simulink model "DealPosLrnd"  (R2018b)
settings: Solver=FixedStepDiscrete  StartTime=0.0  StopTime=10.0  FixedStep=0.01  RelTol=1e-3
undefined symbols (not defined in the file or in its folder): IfKeSMSbSeatMovBkRclnEnable_Val, IfKeSMSbSeatMovBlstOtwdInwdEnable_Val, IfKeSMSbSeatMovCshnFldEnable_Val, IfKeSMSbSeatMovCushnFrtEnable_Val, IfKeSMSbSeatMovFrwdBkwdEnable_Val, IfKeSMSbSeatMovFtrstEnable_Val, IfKeSMSbSeatMovLgrstEnable_Val, IfKeSMSbSeatMovLtwdRtwdEnable_Val, IfVeSMSeStNumConfig, KeSMSbArmscreenMovEnable_Val, KeSMSbIgnorePosLrnd_Val, KeSMSbSeatMovHdFrwdBkwdEnable_Val, KeSMSbSeatMovHdUpwdDnwdEnable_Val, KeSMSbSeatMovLgrstExpdEnable_Val
(part 2 of 2)

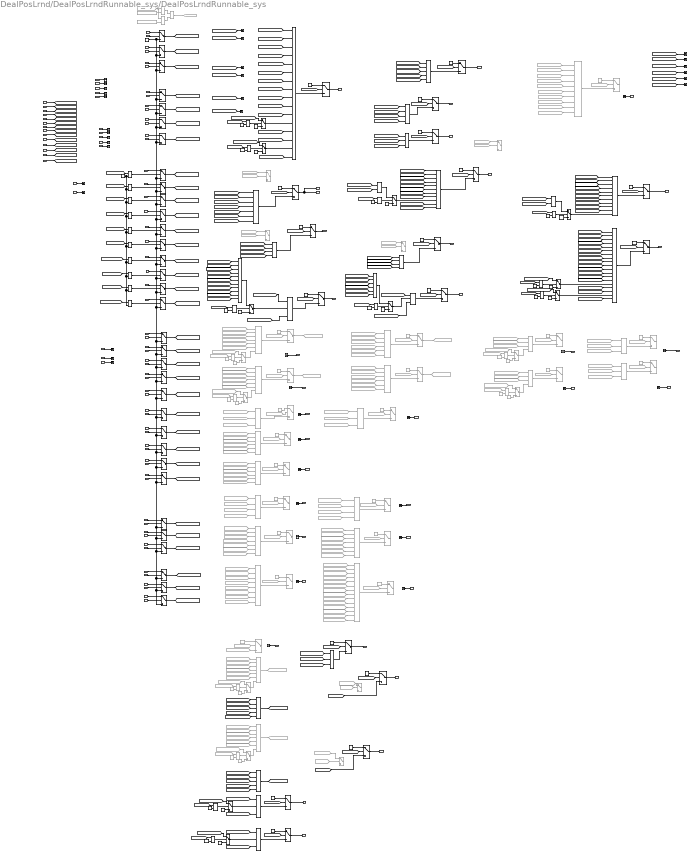
== system DealPosLrnd/DealPosLrndRunnable_sys/DealPosLrndRunnable_sys ==
  note: NOTE:
      | 2023-08-01:新增mode21~26的学习信号，REQ_MSM_607
      | 2023-11-27：四座VIP/全躺/腿托一键打开模式的学习信号，增加前后位置要求。
  note: 四座版本
  note: /* 四座脚踏*/
  note: /*头枕上下*/
  note: /*头枕前后*/
  note: /* 四座腿托伸缩*/
  note: /* 四座脚踏*/
  note: /*头枕前后*/
  note: /* 四座腿托伸缩*/
  note: /*头枕上下*/
  note: 诊断
  note: /*零重力电机*/
  note: /*零重力电机*/
  DrvStBkReclnUpwdDnwdSnsrHmPosLrnd : Inport
  IfVeSMSbDrvStBlstOtwdInwdSnsrHmPosLrnd_Val_read : Inport  Port=2
  IfVeSMSbDrvStCshnFrntUpwdDnwdSnsrHmPosLrnd_Val_read : Inport  Port=3
  IfVeSMSbDrvStCshnRrUpwdDnwdSnsrHmPosLrnd_Val_read : Inport  Port=4
  DrvStFrwdBkwdSnsrHmPosLrnd : Inport  Port=5
  DrvStFtUpwdDnwdSnsrHmPosLrnd : Inport  Port=6
  IfVeSMSbDrvStHdrstUpwdDnwdSnsrHmPosLrnd_Val_read : Inport  Port=7
  IfVeSMSbDrvStLgrstUpwdDnwdSnsrHmPosLrnd_Val_read : Inport  Port=8
  PassStBkReclnUpwdDnwdSnsrHmPosLrnd : Inport  Port=9
  IfVeSMSbPassStBlstOtwdInwdSnsrHmPosLrnd_Val_read : Inport  Port=10
  IfVeSMSbPassStCshnFrntUpwdDnwdSnsrHmPosLrnd_Val_read : Inport  Port=11
  IfVeSMSbPassStCshnRrUpwdDnwdSnsrHmPosLrnd_Val_read : Inport  Port=12
  PassStFrwdBkwdSnsrHmPosLrnd : Inport  Port=13
  PassStFtUpwdDnwdSnsrHmPosLrnd : Inport  Port=14
  IfVeSMSbPassStHdrstUpwdDnwdSnsrHmPosLrnd_Val_read : Inport  Port=15
  IfVeSMSbPassStLgrstUpwdDnwdSnsrHmPosLrnd_Val_read : Inport  Port=16
  SecRwLtStArmScrnSnsrHmPosLrnd : Inport  Port=17
  SecRwLtStBkReclnUpwdDnwdSnsrHmPosLrnd : Inport  Port=18
  SecRwRtStBlstOtwdInwdMovConfig : Inport  Port=19
  IfVeSMSbSecRwLtStBlstOtwdInwdSnsrHmPosLrnd_Val_read : Inport  Port=20
  IfVeSMSbSecRwLtStCshnFrntUpwdDnwdSnsrHmPosLrnd_Val_read : Inport  Port=21
  IfVeSMSbSecRwLtStCshnRrUpwdDnwdSnsrHmPosLrnd_Val_read : Inport  Port=22
  SecRwLtStFrwdBkwdSnsrHmPosLrnd : Inport  Port=23
  SecRwLtStLgrstUpwdDnwdSnsrHmPosLrnd : Inport  Port=24
  SecRwLtStLtwdRtwdSnsrHmPosLrnd : Inport  Port=25
  IfVeSMSbSecRwLtStHdrstUpwdDnwdSnsrHmPosLrnd_Val_read : Inport  Port=26
  IfVeSMSbSecRwRtStArmScrnSnsrHmPosLrnd_Val_read : Inport  Port=27
  SecRwRtStBkReclnUpwdDnwdSnsrHmPosLrnd : Inport  Port=28
  IfVeSMSbSecRwRtStBlstOtwdInwdSnsrHmPosLrnd_Val_read : Inport  Port=29
  IfVeSMSbSecRwRtStCshnFrntUpwdDnwdSnsrHmPosLrnd_Val_read : Inport  Port=30
  IfVeSMSbSecRwRtStCshnRrUpwdDnwdSnsrHmPosLrnd_Val_read : Inport  Port=31
  SecRwRtStFrwdBkwdSnsrHmPosLrnd : Inport  Port=32
  SecRwRtStLgrstUpwdDnwdSnsrHmPosLrnd : Inport  Port=33
  SecRwRtStLtwdRtwdSnsrHmPosLrnd : Inport  Port=34
  IfVeSMSbSecRwRtStHdrstUpwdDnwdSnsrHmPosLrnd_Val_read : Inport  Port=35
  ThdRwLtStBkReclnUpwdDnwdSnsrHmPosLrnd : Inport  Port=36
  ThdRwLtStCshnFldUpwdDnwdSnsrHmPosLrnd : Inport  Port=37
  ThdRwLtStFrwdBkwdSnsrHmPosLrnd : Inport  Port=38
  ThdRwRtStBkReclnUpwdDnwdSnsrHmPosLrnd : Inport  Port=39
  ThdRwRtStCshnFldUpwdDnwdSnsrHmPosLrnd : Inport  Port=40
  ThdRwRtStFrwdBkwdSnsrHmPosLrnd : Inport  Port=41
  KeSMSbSeatMovBkRclnEnable : Inport  Port=42
  KeSMSbSeatMovBlstOtwdInwdEnable : Inport  Port=43
  KeSMSbSeatMovCshnFldEnable : Inport  Port=44
  KeSMSbSeatMovFrwdBkwdEnable : Inport  Port=45
  KeSMSbSeatMovFtrstEnable : Inport  Port=46
  KeSMSbSeatMovLgrstEnable : Inport  Port=47
  KeSMSbSeatMovLtwdRtwdEnable : Inport  Port=48
  KeSMSbIgnorePosLrnd : Inport  Port=49
  KeSMSbArmscreenMovEnable : Inport  Port=50
  DrvStBkReclnUpwdDnwdMovConfig : Inport  Port=51
  DrvStFrwdBkwdMovConfig : Inport  Port=52
  DrvStFtUpwdDnwdMovConfig : Inport  Port=53
  PassStBkReclnUpwdDnwdMovConfig : Inport  Port=54
  PassStFrwdBkwdMovConfig : Inport  Port=55
  PassStFtUpwdDnwdMovConfig : Inport  Port=56
  SecRwRtStBkReclnUpwdDnwdMovConfig : Inport  Port=57
  SecRwRtStFrwdBkwdMovConfig : Inport  Port=58
  SecRwRtStLtwdRtwdMovConfig : Inport  Port=59
  SecRwRtStLgrstUpwdMovConfig : Inport  Port=60
  ThdRwLtStBkReclnUpwdDnwdMovConfig : Inport  Port=61
  ThdRwLtStCshnFldUpwdDnwdMovConfig : Inport  Port=62
  ThdRwLtStFrwdBkwdMovConfig : Inport  Port=63
  ThdRwRtStBkReclnUpwdDnwdMovConfig : Inport  Port=64
  ThdRwRtStCshnFldUpwdDnwdMovConfig : Inport  Port=65
  ThdRwRtStFrwdBkwdMovConfig : Inport  Port=66
  IfVeSMSeStNumConfig : Inport  Port=67
  RrLtStFtUpwdDnwdSnsrHmPosLrnd : Inport  Port=68
  SecRwLtStHdrstFrwdBkwdSnsrHmPosLrnd : Inport  Port=69
  SecRwLtStLgrstOtwdInwdSnsrHmPosLrnd : Inport  Port=70
  RrRtStFtUpwdDnwdSnsrHmPosLrnd : Inport  Port=71
  SecRwRtStHdrstFrwdBkwdSnsrHmPosLrnd : Inport  Port=72
  SecRwRtStLgrstOtwdInwdSnsrHmPosLrnd : Inport  Port=73
  KeSMSbSeatMovHdFrwdBkwdEnable : Inport  Port=74
  KeSMSbSeatMovLgrstExpdEnable : Inport  Port=75
  KeSMSbSeatMovHdUpwdDnwdEnable : Inport  Port=76
  IfVeSMSbRrRtStFtUpwdMovConfig : Inport  Port=77
  IfVeSMSbSecRwRtStHdrstFrwdMovConfig : Inport  Port=78
  IfVeSMSbSecRwRtStLgrstOtwdInwdMovConfig : Inport  Port=79
  IfVeSMSbSecRwRtStHdrstUpwdMovConfig : Inport  Port=80
  IfVeSMSbSecRwRtStArmScrnFrwdBkwdMovConfig : Inport  Port=81
  "IfVeSMSbSecRwRtStCshnFrntUpwdDnwdMovConfig " : Inport  Port=82
  IfKeSMSbSeatMovCushnFrtEnable : Inport  Port=83
  IfVeSMSbPassStFldUpwdDnwdMovConfig : Inport  Port=84
  IfVeSMSbPassStFldUpwdDnwdSnsrHmPosLrnd_Val_read : Inport  Port=85
  AND : Logic  Inputs=16  AllPortsSameDT=off  OutDataTypeStr=boolean
  AND1 : Logic  Commented=on  Inputs=10  AllPortsSameDT=off  OutDataTypeStr=boolean
  AND{6..7,10..11,16,18} (6 alike) : Logic  Inputs=3  AllPortsSameDT=off  OutDataTypeStr=boolean
  AND12 : Logic  AllPortsSameDT=off  OutDataTypeStr=boolean
  AND13 : Logic  Inputs=5  AllPortsSameDT=off  OutDataTypeStr=boolean
  AND14 : Logic  Inputs=11  AllPortsSameDT=off  OutDataTypeStr=boolean
  AND15 : Logic  Inputs=6  AllPortsSameDT=off  OutDataTypeStr=boolean
  AND17 : Logic  Inputs=4  AllPortsSameDT=off  OutDataTypeStr=boolean
  AND19 : Logic  AllPortsSameDT=off  OutDataTypeStr=boolean
  AND2 : Logic  Inputs=7  AllPortsSameDT=off  OutDataTypeStr=boolean
  AND20 : Logic  Inputs=11  AllPortsSameDT=off  OutDataTypeStr=boolean
  AND21 : Logic  Inputs=19  AllPortsSameDT=off  OutDataTypeStr=boolean
  AND3 : Logic  Inputs=11  AllPortsSameDT=off  OutDataTypeStr=boolean
  AND4 : Logic  Inputs=4  AllPortsSameDT=off  OutDataTypeStr=boolean
  AND5 : Logic  Inputs=4  AllPortsSameDT=off  OutDataTypeStr=boolean
  AND8 : Logic  Inputs=5  AllPortsSameDT=off  OutDataTypeStr=boolean
  AND9 : Logic  Inputs=5  AllPortsSameDT=off  OutDataTypeStr=boolean
  Constant{,2..5,13,16,18..19,30,34,37,62..64,67..68} (17 alike) : Constant  Value=true  OutDataTypeStr=boolean
  Constant{1,17,20..24,27..29,40..47,52..53} (20 alike) : Constant  Commented=on  Value=true  OutDataTypeStr=boolean
  Constant{8,10,12,14,26,33,35,66,69,71} (10 alike) : Constant  OutDataTypeStr=uint8
  Constant{7,9,11,25,32,36,65,70,72} (9 alike) : Constant  Value=IfVeSMSeStNumConfig.SeatNum7Config  OutDataTypeStr=Enum: IfVeSMSeStNumConfig
  Constant15 : Constant  Value=IfVeSMSeStNumConfig.SeatNum7Config  OutDataTypeStr=Enum:IfVeSMSeStNumConfig
  Constant31 : Constant  Value=0  OutDataTypeStr=uint8
  Constant38 : Constant  Commented=on  Value=IfVeSMSeStNumConfig.SeatNum4PConfig  OutDataTypeStr=Enum: IfVeSMSeStNumConfig
  Constant39 : Constant  Commented=on  Value=IfVeSMSeStNumConfig.SeatNum4Config  OutDataTypeStr=Enum: IfVeSMSeStNumConfig
  Constant{48,50,54,56,58,60} (6 alike) : Constant  Commented=on  Value=2  OutDataTypeStr=uint8
  Constant{49,51,55,57,59,61} (6 alike) : Constant  Commented=on  OutDataTypeStr=uint8
  Constant6 : Constant  Value=true
  Equal{,1..5,10,25..27} (10 alike) : RelationalOperator  Operator===  OutDataTypeStr=boolean  RndMeth=Simplest
  Equal{6..9,11,13..16,24} (10 alike) : RelationalOperator  Operator=~=  OutDataTypeStr=boolean  RndMeth=Simplest
  Equal{12,17..23} (8 alike) : RelationalOperator  Commented=on  Operator===  OutDataTypeStr=boolean  RndMeth=Simplest
  From{1,11,93,100,109,115,121,164..165,177..178,186,194,202,211,226,234..235,248,252} (20 alike) : From  Commented=on  GotoTag=KeSMSbIgnorePosLrnd
  From{92,101,103,105,131,147} (6 alike) : From  Commented=on  GotoTag=KeSMSeStNum4or4P
  From102 : From  Commented=on  GotoTag=Seat4VIPLtPosLrnd
  From104 : From  Commented=on  GotoTag=Seat4VIPRtPosLrnd
  From106 : From  Commented=on  GotoTag=Seat4RcvyRtPosLrnd
  From{107,112,118,179} (4 alike) : From  Commented=on  GotoTag=SecRwLtStLtwdRtwdSnsrHmPosLrnd
  From{108,114,120,167} (4 alike) : From  Commented=on  GotoTag=SecRwRtStLtwdRtwdSnsrHmPosLrnd
  From110 : From  Commented=on  GotoTag=ThdRwRtStFrwdBkwdSnsrHmPosLrnd
  From{40,111,117,130,166,190,204,213,242,254,258} (11 alike) : From  Commented=on  GotoTag=SecRwLtStFrwdBkwdSnsrHmPosLrnd
  From{45,113,119,168,183,199,208,220,244,256,260} (11 alike) : From  Commented=on  GotoTag=SecRwRtStFrwdBkwdSnsrHmPosLrnd
  From116 : From  Commented=on  GotoTag=ThdRwLtStFrwdBkwdSnsrHmPosLrnd
  From{39,87,124,129,191,203,212,229} (8 alike) : From  Commented=on  GotoTag=SecRwLtStBkReclnUpwdDnwdSnsrHmPosLrnd
  From{41,88,125,174,189,214,230,245} (8 alike) : From  Commented=on  GotoTag=SecRwLtStLgrstUpwdDnwdSnsrHmPosLrnd
  From{89,126,175,188,215,231,246,262} (8 alike) : From  Commented=on  GotoTag=SecRwLtStLgrstOtwdInwdSnsrHmPosLrnd
  From{90,127,176,187,216,232,247} (7 alike) : From  Commented=on  GotoTag=RrLtStFtUpwdDnwdSnsrHmPosLrnd
  From{91,128,139,193,206,218,233} (7 alike) : From  Commented=on  GotoTag=SecRwLtStHdrstUpwdDnwdSnsrHmPosLrnd
  From132 : From  Commented=on  GotoTag=SecRwLtStPosLrnd_Seat4
  From{44,94,134,182,198,207,219,237} (8 alike) : From  Commented=on  GotoTag=SecRwRtStBkReclnUpwdDnwdSnsrHmPosLrnd
  From{46,95,135,171,195,221,238,249} (8 alike) : From  Commented=on  GotoTag=SecRwRtStLgrstUpwdDnwdSnsrHmPosLrnd
  From{96,136,172,197,222,239,250,266} (8 alike) : From  Commented=on  GotoTag=SecRwRtStLgrstOtwdInwdSnsrHmPosLrnd
  From{97,137,173,196,223,240,251} (7 alike) : From  Commented=on  GotoTag=RrRtStFtUpwdDnwdSnsrHmPosLrnd
  From{99,138,185,201,210,225,241} (7 alike) : From  Commented=on  GotoTag=SecRwRtStHdrstUpwdDnwdSnsrHmPosLrnd
  From{140,160,162,192,205,217,228} (7 alike) : From  Commented=on  GotoTag=SecRwLtStHdrstFrwdBkwdSnsrHmPosLrnd
  From148 : From  Commented=on  GotoTag=SecRwRtStPosLrnd_Seat4
  From16 : From  Commented=on  GotoTag=DrvStFtUpwdDnwdSnsrHmPosLrnd
  From{161,163,184,200,209,224,236} (7 alike) : From  Commented=on  GotoTag=SecRwRtStHdrstFrwdBkwdSnsrHmPosLrnd
  From169 : From  Commented=on  GotoTag=ThdRwLtStFrwdBkwdSnsrHmPosLrnd
  From170 : From  Commented=on  GotoTag=ThdRwRtStFrwdBkwdSnsrHmPosLrnd
  From181 : From  Commented=on  GotoTag=IfVeSMSeStNumConfig
  From{227,243,253,255,257,259} (6 alike) : From  Commented=on  GotoTag=KeSMSbSeatMovFrwdBkwdEnable
  From271 : From  Commented=on  GotoTag=SecRwRtStCshnFrntUpwdDnwdSnsrHmPosLrnd
  From49 : From  Commented=on  GotoTag=SecRwLtStCshnFrntUpwdDnwdSnsrHmPosLrnd
  From98 : From  Commented=on  GotoTag=Seat4RcvyLtPosLrnd
  Goto43 : Goto  Commented=on  GotoTag=Seat4VIPLtPosLrnd
  Goto44 : Goto  Commented=on  GotoTag=Seat4VIPRtPosLrnd
  Goto45 : Goto  Commented=on  GotoTag=Seat4RcvyLtPosLrnd
  Goto46 : Goto  Commented=on  GotoTag=Seat4RcvyRtPosLrnd
  Goto47 : Goto  Commented=on  GotoTag=SecRwLtStPosLrnd_Seat4
  Goto49 : Goto  Commented=on  GotoTag=SecRwRtStPosLrnd_Seat4
  Goto51 : Goto  Commented=on  GotoTag=KeSMSeStNum4or4P
  Ground{,5..21} (18 alike) : Ground
  OR{,1,5..6,13..14} (6 alike) : Logic  Commented=on  Inputs=7  AllPortsSameDT=off  OutDataTypeStr=boolean
  OR{2,10,19..20} (4 alike) : Logic  Commented=on  Inputs=3  AllPortsSameDT=off  OutDataTypeStr=boolean
  OR{8..9,11..12} (4 alike) : Logic  Commented=on  Inputs=4  AllPortsSameDT=off  OutDataTypeStr=boolean
  OR15 : Logic  Commented=on  Inputs=8  AllPortsSameDT=off  OutDataTypeStr=boolean
  OR16 : Logic  Commented=on  Inputs=14  AllPortsSameDT=off  OutDataTypeStr=boolean
  OR{3..4,17..18} (4 alike) : Logic  Commented=on  Inputs=6  AllPortsSameDT=off  OutDataTypeStr=boolean
  OR7 : Logic  Commented=on  Operator=OR  AllPortsSameDT=off  OutDataTypeStr=boolean
  Switch{,2..33,35..43,53,55,57..60,64,81..91} (60 alike) : Switch  Criteria=u2 > Threshold
  Switch{1,34,44..52,54,56,61..63,65..80} (32 alike) : Switch  Commented=on  Criteria=u2 > Threshold
  Terminator{,1..26} (27 alike) : Terminator
  IfVeSMSbAcsEntryPosLrnd_Val_write : Outport
  IfVeSMSbAcsExitPosLrnd_Val_write : Outport  Port=2
  IfVeSMSbVIPLtPosLrnd_Val_write : Outport  Port=3
  IfVeSMSbVIPRtPosLrnd_Val_write : Outport  Port=4
  IfVeSMSbRcvyLtPosLrnd_Val_write : Outport  Port=5
  IfVeSMSbRcvyRtPosLrnd_Val_write : Outport  Port=6
  IfVeSMSbLugLtPosLrnd_Val_write : Outport  Port=7
  IfVeSMSbLugRtPosLrnd_Val_write : Outport  Port=8
  IfVeSMSbLyingLtPosLrnd : Outport  Port=9
  IfVeSMSbLyingRtPosLrnd : Outport  Port=10
  IfVeSMSbIntimacyLPosLrnd : Outport  Port=11
  IfVeSMSbFamilyLtPosLrnd : Outport  Port=12
  IfVeSMSbFamilyRtPosLrnd : Outport  Port=13
  IfVeSMSbDrvStPosLrnd_Val_write : Outport  Port=14
  IfVeSMSbPassStPosLrnd_Val_write : Outport  Port=15
  IfVeSMSbSecRwLtStPosLrnd_Val_write : Outport  Port=16
  IfVeSMSbSecRwRtStPosLrnd_Val_write : Outport  Port=17
  IfVeSMSbThdRwLtStPosLrnd_Val_write : Outport  Port=18
  IfVeSMSbThdRwRtStPosLrnd_Val_write : Outport  Port=19
  IfVeSMSbLgrstOpenLtPosLrnd : Outport  Port=20
  IfVeSMSbLgrstCloseLtPosLrnd : Outport  Port=21
  IfVeSMSbLgrstOpenRtPosLrnd : Outport  Port=22
  IfVeSMSbLgrstCloseRtPosLrnd : Outport  Port=23
  IfVeSMSbIntimacyRPosLrnd : Outport  Port=24
  IfVeSMSbAcsEntry4s2LPosLrnd : Outport  Port=25
  IfVeSMSbAcsEntry4s2RPosLrnd : Outport  Port=26
  IfVeSMSbAcsExit4s2LPosLrnd : Outport  Port=27
  IfVeSMSbAcsExit4s2RPosLrnd : Outport  Port=28
  IfVeSMSbAcsEntryAll4sBwdPosLrnd : Outport  Port=29
  IfVeSMSbAcsEntryAll4sFwdPosLrnd : Outport  Port=30
  IfVeSMSbPassReclinerPosLrnd_Val_write : Outport  Port=31
  IfVeSMSbunfold3LPosLrnd_Val_write : Outport  Port=32
  IfVeSMSbunfold3RPosLrnd_Val_write : Outport  Port=33
  IfVeSMSbVIPLtOutPosLrnd_Val_write : Outport  Port=34
  IfVeSMSbVIPRtOutPosLrnd_Val_write : Outport  Port=35
  IfVeSMSbWholeVehMemPosLrnd_Val_write : Outport  Port=36
  wires:
  [KeSMSbIgnorePosLrnd] -> Switch/2
  Switch/1 -> IfVeSMSbAcsEntryPosLrnd_Val_write/1
  Constant/1 -> Switch/1
  From1/1 -> Switch1/2
  Constant1/1 -> Switch1/1
  [KeSMSbIgnorePosLrnd] -> Switch2/2
  Constant2/1 -> Switch2/1
  [KeSMSbIgnorePosLrnd] -> Switch3/2
  Constant3/1 -> Switch3/1
  [KeSMSbIgnorePosLrnd] -> Switch4/2
  Constant4/1 -> Switch4/1
  [KeSMSbIgnorePosLrnd] -> Switch5/2
  Constant5/1 -> Switch5/1
  DrvStBkReclnUpwdDnwdSnsrHmPosLrnd/1 -> Switch6/1
  DrvStFrwdBkwdSnsrHmPosLrnd/1 -> Switch7/1
  DrvStFrwdBkwdMovConfig/1 -> Switch7/2
  DrvStFtUpwdDnwdSnsrHmPosLrnd/1 -> Switch8/1
  PassStBkReclnUpwdDnwdSnsrHmPosLrnd/1 -> Switch9/1
  PassStFrwdBkwdSnsrHmPosLrnd/1 -> Switch10/1
  PassStFtUpwdDnwdSnsrHmPosLrnd/1 -> Switch11/1
  PassStFtUpwdDnwdMovConfig/1 -> Switch11/2
  SecRwLtStBkReclnUpwdDnwdSnsrHmPosLrnd/1 -> Switch12/1
  SecRwLtStFrwdBkwdSnsrHmPosLrnd/1 -> Switch13/1
  SecRwLtStLgrstUpwdDnwdSnsrHmPosLrnd/1 -> Switch14/1
  SecRwLtStLtwdRtwdSnsrHmPosLrnd/1 -> Switch15/1
  SecRwRtStBkReclnUpwdDnwdSnsrHmPosLrnd/1 -> Switch16/1
  SecRwRtStBkReclnUpwdDnwdMovConfig/1 -> Switch16/2
  SecRwRtStFrwdBkwdSnsrHmPosLrnd/1 -> Switch17/1
  SecRwRtStFrwdBkwdMovConfig/1 -> Switch17/2
  SecRwRtStLgrstUpwdMovConfig/1 -> Switch18/2
  SecRwRtStLgrstUpwdDnwdSnsrHmPosLrnd/1 -> Switch18/1
  SecRwRtStLtwdRtwdSnsrHmPosLrnd/1 -> Switch20/1
  SecRwRtStLtwdRtwdMovConfig/1 -> Switch20/2
  ThdRwLtStBkReclnUpwdDnwdSnsrHmPosLrnd/1 -> Switch19/1
  ThdRwLtStBkReclnUpwdDnwdMovConfig/1 -> Switch19/2
  ThdRwLtStCshnFldUpwdDnwdSnsrHmPosLrnd/1 -> Switch21/1
  ThdRwLtStFrwdBkwdSnsrHmPosLrnd/1 -> Switch22/1
  ThdRwRtStBkReclnUpwdDnwdSnsrHmPosLrnd/1 -> Switch23/1
  ThdRwRtStCshnFldUpwdDnwdSnsrHmPosLrnd/1 -> Switch24/1
  ThdRwRtStFrwdBkwdSnsrHmPosLrnd/1 -> Switch25/1
  ThdRwRtStFrwdBkwdMovConfig/1 -> Switch25/2
  KeSMSbSeatMovBkRclnEnable/1 -> [KeSMSbSeatMovBkRclnEnable]
  KeSMSbSeatMovBlstOtwdInwdEnable/1 -> [KeSMSbSeatMovBlstOtwdInwdEnable]
  KeSMSbSeatMovCshnFldEnable/1 -> [KeSMSbSeatMovCshnFldEnable]
  KeSMSbSeatMovFrwdBkwdEnable/1 -> [KeSMSbSeatMovFrwdBkwdEnable]
  KeSMSbSeatMovFtrstEnable/1 -> [KeSMSbSeatMovFtrstEnable]
  KeSMSbSeatMovLgrstEnable/1 -> [KeSMSbSeatMovLgrstEnable]
  KeSMSbSeatMovLtwdRtwdEnable/1 -> [KeSMSbSeatMovLtwdRtwdEnable]
  KeSMSbIgnorePosLrnd/1 -> [KeSMSbIgnorePosLrnd]
  DrvStFtUpwdDnwdMovConfig/1 -> Switch8/2
  PassStBkReclnUpwdDnwdMovConfig/1 -> Switch9/2
  PassStFrwdBkwdMovConfig/1 -> Switch10/2
  ThdRwRtStCshnFldUpwdDnwdMovConfig/1 -> Switch24/2
  IfVeSMSbDrvStLgrstUpwdDnwdSnsrHmPosLrnd_Val_read/1 -> Terminator4/1
  IfVeSMSbDrvStBlstOtwdInwdSnsrHmPosLrnd_Val_read/1 -> Terminator/1
  IfVeSMSbDrvStHdrstUpwdDnwdSnsrHmPosLrnd_Val_read/1 -> Terminator3/1
  IfVeSMSbDrvStCshnFrntUpwdDnwdSnsrHmPosLrnd_Val_read/1 -> Terminator1/1
  IfVeSMSbDrvStCshnRrUpwdDnwdSnsrHmPosLrnd_Val_read/1 -> Terminator2/1
  IfVeSMSbPassStLgrstUpwdDnwdSnsrHmPosLrnd_Val_read/1 -> Terminator9/1
  IfVeSMSbPassStCshnRrUpwdDnwdSnsrHmPosLrnd_Val_read/1 -> Terminator7/1
  IfVeSMSbPassStCshnFrntUpwdDnwdSnsrHmPosLrnd_Val_read/1 -> Terminator6/1
  IfVeSMSbPassStHdrstUpwdDnwdSnsrHmPosLrnd_Val_read/1 -> Terminator8/1
  IfVeSMSbPassStBlstOtwdInwdSnsrHmPosLrnd_Val_read/1 -> Terminator5/1
  IfVeSMSbSecRwLtStBlstOtwdInwdSnsrHmPosLrnd_Val_read/1 -> Terminator11/1
  IfVeSMSbSecRwLtStCshnRrUpwdDnwdSnsrHmPosLrnd_Val_read/1 -> Terminator13/1
  IfVeSMSbSecRwRtStBlstOtwdInwdSnsrHmPosLrnd_Val_read/1 -> Terminator16/1
  IfVeSMSbSecRwRtStCshnRrUpwdDnwdSnsrHmPosLrnd_Val_read/1 -> Terminator18/1
  DrvStBkReclnUpwdDnwdMovConfig/1 -> Switch6/2
  ThdRwLtStCshnFldUpwdDnwdMovConfig/1 -> Switch21/2
  ThdRwLtStFrwdBkwdMovConfig/1 -> Switch22/2
  ThdRwRtStBkReclnUpwdDnwdMovConfig/1 -> Switch23/2
  KeSMSbArmscreenMovEnable/1 -> [KeSMSbArmscreenMovEnable]
  IfVeSMSbSecRwRtStArmScrnSnsrHmPosLrnd_Val_read/1 -> Switch27/1
  SecRwLtStArmScrnSnsrHmPosLrnd/1 -> Switch26/1
  Switch6/1 -> [DrvStBkReclnUpwdDnwdSnsrHmPosLrnd]
  Switch7/1 -> [DrvStFrwdBkwdSnsrHmPosLrnd]
  Switch8/1 -> [DrvStFtUpwdDnwdSnsrHmPosLrnd]
  Switch9/1 -> [PassStBkReclnUpwdDnwdSnsrHmPosLrnd]
  Switch10/1 -> [PassStFrwdBkwdSnsrHmPosLrnd]
  Switch11/1 -> [PassStFtUpwdDnwdSnsrHmPosLrnd]
  Switch12/1 -> [SecRwLtStBkReclnUpwdDnwdSnsrHmPosLrnd]
  Switch13/1 -> [SecRwLtStFrwdBkwdSnsrHmPosLrnd]
  Switch14/1 -> [SecRwLtStLgrstUpwdDnwdSnsrHmPosLrnd]
  Switch15/1 -> [SecRwLtStLtwdRtwdSnsrHmPosLrnd]
  Switch26/1 -> [SecRwLtStArmScrnSnsrHmPosLrnd]
  Switch16/1 -> [SecRwRtStBkReclnUpwdDnwdSnsrHmPosLrnd]
  Switch17/1 -> [SecRwRtStFrwdBkwdSnsrHmPosLrnd]
  Switch18/1 -> [SecRwRtStLgrstUpwdDnwdSnsrHmPosLrnd]
  Switch20/1 -> [SecRwRtStLtwdRtwdSnsrHmPosLrnd]
  Switch27/1 -> [SecRwRtStArmScrnSnsrHmPosLrnd]
  Switch19/1 -> [ThdRwLtStBkReclnUpwdDnwdSnsrHmPosLrnd]
  Switch21/1 -> [ThdRwLtStCshnFldUpwdDnwdSnsrHmPosLrnd]
  Switch22/1 -> [ThdRwLtStFrwdBkwdSnsrHmPosLrnd]
  Switch23/1 -> [ThdRwRtStBkReclnUpwdDnwdSnsrHmPosLrnd]
  Switch24/1 -> [ThdRwRtStCshnFldUpwdDnwdSnsrHmPosLrnd]
  Switch25/1 -> [ThdRwRtStFrwdBkwdSnsrHmPosLrnd]
  IfVeSMSeStNumConfig/1 -> [IfVeSMSeStNumConfig]
  [IfVeSMSeStNumConfig] -> Equal/1
  Constant7/1 -> Equal/2
  Equal/1 -> Switch28/2
  [ThdRwLtStCshnFldUpwdDnwdSnsrHmPosLrnd] -> Switch28/1
  Constant8/1 -> Switch28/3
  Constant10/1 -> Switch29/3
  Equal1/1 -> Switch29/2
  Constant9/1 -> Equal1/2
  [IfVeSMSeStNumConfig] -> Equal1/1
  [ThdRwRtStCshnFldUpwdDnwdSnsrHmPosLrnd] -> Switch29/1
  AND/1 -> Switch/3
  AND1/1 -> Switch1/3
  [SecRwLtStBkReclnUpwdDnwdSnsrHmPosLrnd] -> AND4/1
  [SecRwLtStLgrstUpwdDnwdSnsrHmPosLrnd] -> AND4/2
  [SecRwRtStBkReclnUpwdDnwdSnsrHmPosLrnd] -> AND5/1
  [SecRwRtStLgrstUpwdDnwdSnsrHmPosLrnd] -> AND5/2
  [ThdRwLtStFrwdBkwdSnsrHmPosLrnd] -> AND6/3
  Switch30/1 -> AND6/2
  Constant12/1 -> Switch30/3
  [ThdRwLtStBkReclnUpwdDnwdSnsrHmPosLrnd] -> AND6/1
  Equal2/1 -> Switch30/2
  [IfVeSMSeStNumConfig] -> Equal2/1
  Constant11/1 -> Equal2/2
  Constant13/1 -> Switch31/1
  [KeSMSbIgnorePosLrnd] -> Switch31/2
  AND6/1 -> Switch31/3
  [IfVeSMSeStNumConfig] -> Equal3/1
  Constant15/1 -> Equal3/2
  Equal3/1 -> Switch32/2
  Constant14/1 -> Switch32/3
  Switch32/1 -> AND7/2
  [ThdRwRtStFrwdBkwdSnsrHmPosLrnd] -> AND7/3
  Constant16/1 -> Switch33/1
  [KeSMSbIgnorePosLrnd] -> Switch33/2
  AND7/1 -> Switch33/3
  [ThdRwLtStBkReclnUpwdDnwdSnsrHmPosLrnd] -> AND2/6
  [ThdRwLtStFrwdBkwdSnsrHmPosLrnd] -> AND2/7
  KeSMSbSeatMovHdFrwdBkwdEnable/1 -> [KeSMSbSeatMovHdFrwdBkwdEnable]
  KeSMSbSeatMovLgrstExpdEnable/1 -> [KeSMSbSeatMovLgrstExpdEnable]
  RrLtStFtUpwdDnwdSnsrHmPosLrnd/1 -> Switch36/1
  Switch36/1 -> [RrLtStFtUpwdDnwdSnsrHmPosLrnd]
  IfVeSMSbSecRwLtStHdrstUpwdDnwdSnsrHmPosLrnd_Val_read/1 -> Switch37/1
  Switch37/1 -> [SecRwLtStHdrstUpwdDnwdSnsrHmPosLrnd]
  SecRwLtStHdrstFrwdBkwdSnsrHmPosLrnd/1 -> Switch38/1
  Switch38/1 -> [SecRwLtStHdrstFrwdBkwdSnsrHmPosLrnd]
  SecRwLtStLgrstOtwdInwdSnsrHmPosLrnd/1 -> Switch39/1
  Switch39/1 -> [SecRwLtStLgrstOtwdInwdSnsrHmPosLrnd]
  KeSMSbSeatMovHdUpwdDnwdEnable/1 -> [KeSMSbSeatMovHdUpwdDnwdEnable]
  IfVeSMSbRrRtStFtUpwdMovConfig/1 -> Switch40/2
  RrRtStFtUpwdDnwdSnsrHmPosLrnd/1 -> Switch40/1
  Switch40/1 -> [RrRtStFtUpwdDnwdSnsrHmPosLrnd]
  IfVeSMSbSecRwRtStHdrstFrwdMovConfig/1 -> Switch41/2
  SecRwRtStHdrstFrwdBkwdSnsrHmPosLrnd/1 -> Switch41/1
  Switch41/1 -> [SecRwRtStHdrstFrwdBkwdSnsrHmPosLrnd]
  IfVeSMSbSecRwRtStLgrstOtwdInwdMovConfig/1 -> Switch42/2
  SecRwRtStLgrstOtwdInwdSnsrHmPosLrnd/1 -> Switch42/1
  Switch42/1 -> [SecRwRtStLgrstOtwdInwdSnsrHmPosLrnd]
  IfVeSMSbSecRwRtStHdrstUpwdDnwdSnsrHmPosLrnd_Val_read/1 -> Switch43/1
  Constant6/1 -> Switch7/3, Switch83/3, Switch12/3, Switch13/3, Switch15/3, Switch26/3, Switch36/3, Switch37/3, Switch38/3, Switch39/3, Switch81/3, Switch16/3, Switch17/3, Switch18/3, Switch20/3, Switch27/3, Switch40/3, Switch41/3, Switch42/3, Switch43/3, Switch82/3, Switch23/3, Switch24/3, Switch25/3, Switch22/3, Switch21/3, Switch19/3, Switch14/3, Switch11/3, Switch10/3, Switch9/3, Switch8/3, Switch6/3
  IfVeSMSbSecRwRtStHdrstUpwdMovConfig/1 -> Switch43/2
  Switch43/1 -> [SecRwRtStHdrstUpwdDnwdSnsrHmPosLrnd]
  From87/1 -> OR/1
  From88/1 -> OR/2
  From89/1 -> OR/3
  From90/1 -> OR/4
  From91/1 -> OR/5
  From93/1 -> Switch44/2
  Constant21/1 -> Switch44/1
  OR/1 -> Switch44/3
  Switch44/1 -> Goto43/1
  From94/1 -> OR1/1
  From95/1 -> OR1/2
  From96/1 -> OR1/3
  From97/1 -> OR1/4
  Constant22/1 -> Switch45/1
  From100/1 -> Switch45/2
  OR1/1 -> Switch45/3
  Switch45/1 -> Goto44/1
  From102/1 -> Switch46/1
  From103/1 -> Switch47/2
  From99/1 -> OR1/5
  From104/1 -> Switch47/1
  From98/1 -> Switch48/1
  From105/1 -> Switch49/2
  From106/1 -> Switch49/1
  OR2/1 -> Switch50/3
  From109/1 -> Switch50/2
  Constant27/1 -> Switch50/1
  Constant28/1 -> Switch51/1
  From115/1 -> Switch51/2
  OR3/1 -> Switch51/3
  From121/1 -> Switch52/2
  Constant29/1 -> Switch52/1
  OR4/1 -> Switch52/3
  Switch4/1 -> IfVeSMSbRcvyLtPosLrnd_Val_write/1
  Switch5/1 -> IfVeSMSbRcvyRtPosLrnd_Val_write/1
  From11/1 -> Switch34/2
  Constant17/1 -> Switch34/1
  From16/1 -> Switch34/3
  Constant18/1 -> Switch35/1
  [KeSMSbIgnorePosLrnd] -> Switch35/2
  AND16/1 -> Switch35/3
  [SecRwLtStBkReclnUpwdDnwdSnsrHmPosLrnd] -> AND8/1
  [SecRwLtStFrwdBkwdSnsrHmPosLrnd] -> AND8/2
  [SecRwLtStLgrstUpwdDnwdSnsrHmPosLrnd] -> AND8/3
  [SecRwLtStLgrstOtwdInwdSnsrHmPosLrnd] -> AND8/4
  Constant19/1 -> Switch53/1
  [KeSMSbIgnorePosLrnd] -> Switch53/2
  From125/1 -> OR5/2
  From126/1 -> OR5/3
  From128/1 -> OR5/5
  From124/1 -> OR5/1
  From127/1 -> OR5/4
  AND8/1 -> [SecRwLtStPosLrnd_Seat6_7]
  From132/1 -> Switch54/1
  Switch53/1 -> IfVeSMSbSecRwLtStPosLrnd_Val_write/1
  From134/1 -> OR6/1
  From135/1 -> OR6/2
  From136/1 -> OR6/3
  From137/1 -> OR6/4
  From138/1 -> OR6/5
  OR6/1 -> Goto49/1
  [SecRwRtStCshnFrntUpwdDnwdSnsrHmPosLrnd] -> AND9/5
  [SecRwRtStBkReclnUpwdDnwdSnsrHmPosLrnd] -> AND9/1
  [SecRwRtStFrwdBkwdSnsrHmPosLrnd] -> AND9/2
  [SecRwRtStLgrstUpwdDnwdSnsrHmPosLrnd] -> AND9/3
  [SecRwRtStLgrstOtwdInwdSnsrHmPosLrnd] -> AND9/4
  AND9/1 -> [SecRwRtStPosLrnd_Seat6_7]
  [KeSMSbIgnorePosLrnd] -> Switch55/2
  Constant30/1 -> Switch55/1
  From148/1 -> Switch56/1
  From147/1 -> Switch56/2
  Switch55/1 -> IfVeSMSbSecRwRtStPosLrnd_Val_write/1
  Constant33/1 -> Switch57/3
  [ThdRwLtStCshnFldUpwdDnwdSnsrHmPosLrnd] -> Switch57/1
  Equal5/1 -> Switch57/2
  [IfVeSMSeStNumConfig] -> Equal5/1
  Constant32/1 -> Equal5/2
  Constant34/1 -> Switch58/1
  AND10/1 -> Switch58/3
  [KeSMSbIgnorePosLrnd] -> Switch58/2
  [ThdRwLtStBkReclnUpwdDnwdSnsrHmPosLrnd] -> AND10/1
  Switch57/1 -> AND10/2
  [ThdRwLtStFrwdBkwdSnsrHmPosLrnd] -> AND10/3
  Switch58/1 -> IfVeSMSbThdRwLtStPosLrnd_Val_write/1
  Constant36/1 -> Equal10/2
  Equal10/1 -> Switch59/2
  [IfVeSMSeStNumConfig] -> Equal10/1
  [ThdRwRtStCshnFldUpwdDnwdSnsrHmPosLrnd] -> Switch59/1
  Constant35/1 -> Switch59/3
  [ThdRwRtStBkReclnUpwdDnwdSnsrHmPosLrnd] -> AND11/1
  [ThdRwRtStFrwdBkwdSnsrHmPosLrnd] -> AND11/3
  Switch59/1 -> AND11/2
  [KeSMSbIgnorePosLrnd] -> Switch60/2
  Constant37/1 -> Switch60/1
  AND11/1 -> Switch60/3
  Switch60/1 -> IfVeSMSbThdRwRtStPosLrnd_Val_write/1
  OR5/1 -> Goto47/1
  From160/1 -> OR/6
  From161/1 -> OR1/6
  From162/1 -> OR5/6
  From163/1 -> OR6/6
  Constant38/1 -> Equal17/2
  OR7/1 -> Goto51/1
  Equal17/1 -> OR7/2
  Constant39/1 -> Equal12/2
  Equal12/1 -> OR7/1
  From181/1 -> Equal17/1, Equal12/1
  From101/1 -> Switch46/2
  From92/1 -> Switch48/2
  From131/1 -> Switch54/2
  From166/1 -> OR2/1
  From107/1 -> OR2/2
  From169/1 -> OR3/1
  From110/1 -> OR3/2
  From111/1 -> OR3/3
  From112/1 -> OR3/4
  From113/1 -> OR3/5
  From114/1 -> OR3/6
  From170/1 -> OR4/1
  From116/1 -> OR4/2
  From117/1 -> OR4/3
  From118/1 -> OR4/4
  From119/1 -> OR4/5
  From120/1 -> OR4/6
  From174/1 -> OR8/1
  From176/1 -> OR8/3
  From175/1 -> OR8/2
  Constant20/1 -> Switch61/1
  From177/1 -> Switch61/2
  OR8/1 -> Switch61/3
  OR9/1 -> Switch62/3
  From178/1 -> Switch62/2
  Constant23/1 -> Switch62/1
  From173/1 -> OR9/3
  From172/1 -> OR9/2
  From171/1 -> OR9/1
  From108/1 -> OR2/3
  Constant24/1 -> Switch63/1
  From165/1 -> Switch63/2
  OR10/1 -> Switch63/3
  From168/1 -> OR10/1
  From167/1 -> OR10/2
  From179/1 -> OR10/3
  Constant25/1 -> Equal4/2
  Equal4/1 -> Switch64/2
  [IfVeSMSeStNumConfig] -> Equal4/1
  Constant26/1 -> Switch64/3
  AND12/1 -> Switch64/1
  [ThdRwLtStBkReclnUpwdDnwdSnsrHmPosLrnd] -> AND12/1
  [ThdRwLtStFrwdBkwdSnsrHmPosLrnd] -> AND12/2
  [KeSMSbSeatMovBkRclnEnable] -> Equal6/1
  Constant31/1 -> Equal15/2, Equal24/2, Equal16/2, Equal14/2, Equal13/2, Equal11/2, Equal9/2, Equal8/2, Equal7/2, Equal6/2
  Equal6/1 -> Switch12/2
  [KeSMSbSeatMovFrwdBkwdEnable] -> Equal7/1
  Equal7/1 -> Switch13/2
  [KeSMSbSeatMovLgrstEnable] -> Equal8/1
  Equal8/1 -> Switch14/2
  Equal9/1 -> Switch15/2
  [KeSMSbSeatMovLtwdRtwdEnable] -> Equal9/1
  Equal11/1 -> Switch26/2
  [KeSMSbArmscreenMovEnable] -> Equal11/1
  Equal13/1 -> Switch36/2
  [KeSMSbSeatMovFtrstEnable] -> Equal13/1
  Equal14/1 -> Switch37/2
  [KeSMSbSeatMovHdUpwdDnwdEnable] -> Equal14/1
  Equal15/1 -> Switch38/2
  [KeSMSbSeatMovHdFrwdBkwdEnable] -> Equal15/1
  Equal16/1 -> Switch39/2
  [KeSMSbSeatMovLgrstExpdEnable] -> Equal16/1
  From130/1 -> OR11/2
  From129/1 -> OR11/1
  From164/1 -> Switch65/2
  OR11/1 -> Switch65/3
  Constant40/1 -> Switch65/1
  From182/1 -> OR12/1
  From183/1 -> OR12/2
  From185/1 -> OR12/4
  From184/1 -> OR12/3
  OR12/1 -> Switch66/3
  From186/1 -> Switch66/2
  Constant41/1 -> Switch66/1
  From140/1 -> OR11/3
  From139/1 -> OR11/4
  From191/1 -> OR13/1
  From190/1 -> OR13/2
  From189/1 -> OR13/3
  From188/1 -> OR13/4
  From187/1 -> OR13/5
  From192/1 -> OR13/6
  From193/1 -> OR13/7
  From194/1 -> Switch67/2
  OR13/1 -> Switch67/3
  Constant42/1 -> Switch67/1
  From198/1 -> OR14/1
  From199/1 -> OR14/2
  From195/1 -> OR14/3
  From197/1 -> OR14/4
  From196/1 -> OR14/5
  From200/1 -> OR14/6
  From201/1 -> OR14/7
  OR14/1 -> Switch68/3
  From202/1 -> Switch68/2
  Constant43/1 -> Switch68/1
  From203/1 -> OR15/1
  From204/1 -> OR15/2
  From205/1 -> OR15/3
  From206/1 -> OR15/4
  From207/1 -> OR15/5
  From208/1 -> OR15/6
  From209/1 -> OR15/7
  From210/1 -> OR15/8
  From211/1 -> Switch69/2
  Constant44/1 -> Switch69/1
  OR15/1 -> Switch69/3
  From212/1 -> OR16/1
  From213/1 -> OR16/2
  From214/1 -> OR16/3
  From215/1 -> OR16/4
  From216/1 -> OR16/5
  From217/1 -> OR16/6
  From218/1 -> OR16/7
  From219/1 -> OR16/8
  From220/1 -> OR16/9
  From221/1 -> OR16/10
  From222/1 -> OR16/11
  From223/1 -> OR16/12
  From224/1 -> OR16/13
  From225/1 -> OR16/14
  From226/1 -> Switch70/2
  OR16/1 -> Switch70/3
  Constant45/1 -> Switch70/1
  IfVeSMSbSecRwRtStArmScrnFrwdBkwdMovConfig/1 -> Switch27/2
  SecRwRtStBlstOtwdInwdMovConfig/1 -> Terminator10/1
  From232/1 -> OR17/4
  From231/1 -> OR17/3
  From230/1 -> OR17/2
  From233/1 -> OR17/5
  Constant46/1 -> Switch71/1
  From234/1 -> Switch71/2
  OR17/1 -> Switch71/3
  From229/1 -> OR17/1
  From228/1 -> OR17/6
  From241/1 -> OR18/5
  From236/1 -> OR18/6
  From238/1 -> OR18/2
  From239/1 -> OR18/3
  From240/1 -> OR18/4
  OR18/1 -> Switch72/3
  From237/1 -> OR18/1
  From235/1 -> Switch72/2
  Constant47/1 -> Switch72/1
  Switch71/1 -> Goto45/1
  Switch72/1 -> Goto46/1
  From227/1 -> Equal18/1
  Constant48/1 -> Equal18/2
  Equal18/1 -> Switch73/2
  From242/1 -> Switch73/1
  Constant49/1 -> Switch73/3
  Switch73/1 -> OR/7
  Constant51/1 -> Switch74/3
  Equal19/1 -> Switch74/2
  Constant50/1 -> Equal19/2
  From243/1 -> Equal19/1
  From244/1 -> Switch74/1
  Switch74/1 -> OR1/7
  OR19/1 -> Switch75/3
  From248/1 -> Switch75/2
  Constant52/1 -> Switch75/1
  From246/1 -> OR19/2
  From247/1 -> OR19/3
  From245/1 -> OR19/1
  From249/1 -> OR20/1
  From250/1 -> OR20/2
  From251/1 -> OR20/3
  Constant53/1 -> Switch76/1
  From252/1 -> Switch76/2
  OR20/1 -> Switch76/3
  Constant55/1 -> Switch77/3
  From254/1 -> Switch77/1
  Equal20/1 -> Switch77/2
  Constant54/1 -> Equal20/2
  From253/1 -> Equal20/1
  Switch77/1 -> OR8/4
  From256/1 -> Switch78/1
  From255/1 -> Equal21/1
  Constant56/1 -> Equal21/2
  Equal21/1 -> Switch78/2
  Constant57/1 -> Switch78/3
  Switch78/1 -> OR9/4
  Constant59/1 -> Switch79/3
  From258/1 -> Switch79/1
  Equal22/1 -> Switch79/2
  Constant58/1 -> Equal22/2
  From257/1 -> Equal22/1
  Switch79/1 -> OR5/7
  From260/1 -> Switch80/1
  From259/1 -> Equal23/1
  Constant60/1 -> Equal23/2
  Equal23/1 -> Switch80/2
  Constant61/1 -> Switch80/3
  Switch80/1 -> OR6/7
  [DrvStFtUpwdDnwdSnsrHmPosLrnd] -> Terminator14/1
  [PassStFtUpwdDnwdSnsrHmPosLrnd] -> Terminator15/1
  [SecRwLtStLtwdRtwdSnsrHmPosLrnd] -> Terminator19/1
  [SecRwLtStArmScrnSnsrHmPosLrnd] -> Terminator20/1
  [SecRwRtStLtwdRtwdSnsrHmPosLrnd] -> Terminator21/1
  [SecRwRtStArmScrnSnsrHmPosLrnd] -> Terminator22/1
  [IfKeSMSbSeatMovCushnFrtEnable] -> Equal24/1
  Equal24/1 -> Switch81/2
  Switch81/1 -> [SecRwLtStCshnFrntUpwdDnwdSnsrHmPosLrnd]
  IfVeSMSbSecRwLtStCshnFrntUpwdDnwdSnsrHmPosLrnd_Val_read/1 -> Switch81/1
  "IfVeSMSbSecRwRtStCshnFrntUpwdDnwdMovConfig "/1 -> Switch82/2
  Switch82/1 -> [SecRwRtStCshnFrntUpwdDnwdSnsrHmPosLrnd]
  [SecRwLtStBkReclnUpwdDnwdSnsrHmPosLrnd] -> AND/1
  [SecRwLtStFrwdBkwdSnsrHmPosLrnd] -> AND/2
  [SecRwLtStLgrstUpwdDnwdSnsrHmPosLrnd] -> AND/3
  [SecRwLtStLgrstOtwdInwdSnsrHmPosLrnd] -> AND/4
  [SecRwLtStCshnFrntUpwdDnwdSnsrHmPosLrnd] -> AND/5
  [SecRwRtStBkReclnUpwdDnwdSnsrHmPosLrnd] -> AND/6
  [SecRwRtStFrwdBkwdSnsrHmPosLrnd] -> AND/7
  [SecRwRtStLgrstUpwdDnwdSnsrHmPosLrnd] -> AND/8
  [SecRwRtStLgrstOtwdInwdSnsrHmPosLrnd] -> AND/9
  [SecRwRtStCshnFrntUpwdDnwdSnsrHmPosLrnd] -> AND/10
  [ThdRwLtStBkReclnUpwdDnwdSnsrHmPosLrnd] -> AND/11
  Switch28/1 -> AND/12
  [ThdRwLtStFrwdBkwdSnsrHmPosLrnd] -> AND/13
  [ThdRwRtStBkReclnUpwdDnwdSnsrHmPosLrnd] -> AND/14
  Switch29/1 -> AND/15
  [ThdRwRtStFrwdBkwdSnsrHmPosLrnd] -> AND/16
  [SecRwLtStLgrstOtwdInwdSnsrHmPosLrnd] -> AND4/3
  [SecRwLtStCshnFrntUpwdDnwdSnsrHmPosLrnd] -> AND4/4
  [SecRwRtStLgrstOtwdInwdSnsrHmPosLrnd] -> AND5/3
  [SecRwRtStCshnFrntUpwdDnwdSnsrHmPosLrnd] -> AND5/4
  IfVeSMSbSecRwRtStCshnFrntUpwdDnwdSnsrHmPosLrnd_Val_read/1 -> Switch82/1
  IfKeSMSbSeatMovCushnFrtEnable/1 -> [IfKeSMSbSeatMovCushnFrtEnable]
  [DrvStFtUpwdDnwdSnsrHmPosLrnd] -> Terminator12/1
  [PassStFtUpwdDnwdSnsrHmPosLrnd] -> Terminator17/1
  [SecRwLtStLtwdRtwdSnsrHmPosLrnd] -> Terminator23/1
  [SecRwLtStArmScrnSnsrHmPosLrnd] -> Terminator24/1
  From39/1 -> AND1/1
  From40/1 -> AND1/2
  From41/1 -> AND1/3
  From262/1 -> AND1/4
  From49/1 -> AND1/5
  From44/1 -> AND1/6
  From45/1 -> AND1/7
  From46/1 -> AND1/8
  From271/1 -> AND1/10
  From266/1 -> AND1/9
  [SecRwRtStLtwdRtwdSnsrHmPosLrnd] -> Terminator25/1
  [SecRwRtStArmScrnSnsrHmPosLrnd] -> Terminator26/1
  Ground/1 -> IfVeSMSbAcsExitPosLrnd_Val_write/1
  Ground5/1 -> IfVeSMSbLyingLtPosLrnd/1
  Ground6/1 -> IfVeSMSbLyingRtPosLrnd/1
  Ground7/1 -> IfVeSMSbLgrstOpenLtPosLrnd/1
  Ground8/1 -> IfVeSMSbLgrstCloseLtPosLrnd/1
  Ground9/1 -> IfVeSMSbLgrstOpenRtPosLrnd/1
  Ground10/1 -> IfVeSMSbLgrstCloseRtPosLrnd/1
  Ground11/1 -> IfVeSMSbIntimacyLPosLrnd/1
  Ground12/1 -> IfVeSMSbIntimacyRPosLrnd/1
  Ground13/1 -> IfVeSMSbFamilyLtPosLrnd/1
  Ground14/1 -> IfVeSMSbFamilyRtPosLrnd/1
  Ground15/1 -> IfVeSMSbAcsEntry4s2LPosLrnd/1
  Ground16/1 -> IfVeSMSbAcsEntry4s2RPosLrnd/1
  Ground17/1 -> IfVeSMSbAcsExit4s2LPosLrnd/1
  Ground18/1 -> IfVeSMSbAcsExit4s2RPosLrnd/1
  Ground19/1 -> IfVeSMSbAcsEntryAll4sBwdPosLrnd/1
  Ground20/1 -> IfVeSMSbAcsEntryAll4sFwdPosLrnd/1
  Ground21/1 -> IfVeSMSbDrvStPosLrnd_Val_write/1
  [SecRwLtStCshnFrntUpwdDnwdSnsrHmPosLrnd] -> AND8/5
  AND4/1 -> Switch4/3
  AND5/1 -> Switch5/3
  [SecRwLtStPosLrnd_Seat6_7] -> Switch53/3
  [SecRwRtStPosLrnd_Seat6_7] -> Switch55/3
  IfVeSMSbPassStFldUpwdDnwdMovConfig/1 -> Switch83/2
  IfVeSMSbPassStFldUpwdDnwdSnsrHmPosLrnd_Val_read/1 -> Switch83/1
  Switch83/1 -> [PassStFldUpwdDnwdSnsrHmPosLrnd]
  [PassStBkReclnUpwdDnwdSnsrHmPosLrnd] -> AND13/2
  [PassStFldUpwdDnwdSnsrHmPosLrnd] -> AND13/3
  [PassStFrwdBkwdSnsrHmPosLrnd] -> AND13/1
  AND13/1 -> Switch84/3
  [KeSMSbIgnorePosLrnd] -> Switch84/2
  Constant62/1 -> Switch84/1
  Switch84/1 -> IfVeSMSbPassReclinerPosLrnd_Val_write/1
  [SecRwLtStBkReclnUpwdDnwdSnsrHmPosLrnd] -> AND2/1
  [SecRwLtStFrwdBkwdSnsrHmPosLrnd] -> AND2/2
  [SecRwLtStLgrstUpwdDnwdSnsrHmPosLrnd] -> AND2/3
  [SecRwLtStLgrstOtwdInwdSnsrHmPosLrnd] -> AND2/4
  [SecRwLtStCshnFrntUpwdDnwdSnsrHmPosLrnd] -> AND2/5
  Switch3/1 -> IfVeSMSbVIPRtPosLrnd_Val_write/1
  Switch31/1 -> IfVeSMSbLugLtPosLrnd_Val_write/1
  AND14/1 -> Switch30/1
  Switch33/1 -> IfVeSMSbLugRtPosLrnd_Val_write/1
  [ThdRwRtStBkReclnUpwdDnwdSnsrHmPosLrnd] -> AND7/1
  AND15/1 -> Switch32/1
  Switch35/1 -> IfVeSMSbPassStPosLrnd_Val_write/1
  [PassStFrwdBkwdSnsrHmPosLrnd] -> AND16/1
  [PassStBkReclnUpwdDnwdSnsrHmPosLrnd] -> AND16/2
  [PassStFldUpwdDnwdSnsrHmPosLrnd] -> AND16/3
  Constant63/1 -> Switch85/1
  [KeSMSbIgnorePosLrnd] -> Switch85/2
  [SecRwLtStBkReclnUpwdDnwdSnsrHmPosLrnd] -> AND17/1
  [SecRwRtStBkReclnUpwdDnwdSnsrHmPosLrnd] -> AND17/2
  [ThdRwLtStBkReclnUpwdDnwdSnsrHmPosLrnd] -> AND17/3
  [ThdRwLtStCshnFldUpwdDnwdSnsrHmPosLrnd] -> AND17/4
  AND17/1 -> Switch85/3
  Switch85/1 -> IfVeSMSbunfold3LPosLrnd_Val_write/1
  [ThdRwRtStBkReclnUpwdDnwdSnsrHmPosLrnd] -> AND18/1
  [ThdRwRtStCshnFldUpwdDnwdSnsrHmPosLrnd] -> AND18/2
  [SecRwRtStBkReclnUpwdDnwdSnsrHmPosLrnd] -> AND18/3
  AND18/1 -> Switch86/3
  [KeSMSbIgnorePosLrnd] -> Switch86/2
  Constant64/1 -> Switch86/1
  Switch86/1 -> IfVeSMSbunfold3RPosLrnd_Val_write/1
  AND3/1 -> Switch3/3
  AND2/1 -> Switch2/3
  [ThdRwLtStFrwdBkwdSnsrHmPosLrnd] -> AND19/2
  [ThdRwLtStBkReclnUpwdDnwdSnsrHmPosLrnd] -> AND19/1
  AND19/1 -> Switch87/1
  Constant66/1 -> Switch87/3
  [IfVeSMSeStNumConfig] -> Equal25/1
  Equal25/1 -> Switch87/2
  Constant65/1 -> Equal25/2
  Switch87/1 -> AND20/11
  [ThdRwRtStFrwdBkwdSnsrHmPosLrnd] -> AND20/10
  [ThdRwRtStBkReclnUpwdDnwdSnsrHmPosLrnd] -> AND20/9
  [SecRwRtStCshnFrntUpwdDnwdSnsrHmPosLrnd] -> AND20/8
  [SecRwRtStLgrstOtwdInwdSnsrHmPosLrnd] -> AND20/7
  [SecRwRtStLgrstUpwdDnwdSnsrHmPosLrnd] -> AND20/6
  [SecRwRtStFrwdBkwdSnsrHmPosLrnd] -> AND20/5
  [SecRwRtStBkReclnUpwdDnwdSnsrHmPosLrnd] -> AND20/4
  [PassStFldUpwdDnwdSnsrHmPosLrnd] -> AND20/3
  [PassStBkReclnUpwdDnwdSnsrHmPosLrnd] -> AND20/2
  [PassStFrwdBkwdSnsrHmPosLrnd] -> AND20/1
  Constant67/1 -> Switch88/1
  [KeSMSbIgnorePosLrnd] -> Switch88/2
  AND20/1 -> Switch88/3
  Switch88/1 -> IfVeSMSbVIPRtOutPosLrnd_Val_write/1
  Switch2/1 -> IfVeSMSbVIPLtOutPosLrnd_Val_write/1, IfVeSMSbVIPLtPosLrnd_Val_write/1
  [SecRwRtStBkReclnUpwdDnwdSnsrHmPosLrnd] -> AND3/1
  [SecRwRtStFrwdBkwdSnsrHmPosLrnd] -> AND3/2
  [SecRwRtStLgrstUpwdDnwdSnsrHmPosLrnd] -> AND3/3
  [SecRwRtStLgrstOtwdInwdSnsrHmPosLrnd] -> AND3/4
  [SecRwRtStCshnFrntUpwdDnwdSnsrHmPosLrnd] -> AND3/5
  [PassStBkReclnUpwdDnwdSnsrHmPosLrnd] -> AND3/6
  [PassStFldUpwdDnwdSnsrHmPosLrnd] -> AND3/7
  [PassStFrwdBkwdSnsrHmPosLrnd] -> AND3/8
  [ThdRwRtStBkReclnUpwdDnwdSnsrHmPosLrnd] -> AND3/10
  [ThdRwRtStFrwdBkwdSnsrHmPosLrnd] -> AND3/11
  Switch64/1 -> AND3/9
  [SecRwLtStBkReclnUpwdDnwdSnsrHmPosLrnd] -> AND14/1
  [SecRwLtStFrwdBkwdSnsrHmPosLrnd] -> AND14/2
  [SecRwLtStCshnFrntUpwdDnwdSnsrHmPosLrnd] -> AND14/3
  [SecRwLtStLgrstOtwdInwdSnsrHmPosLrnd] -> AND14/4
  [SecRwLtStLgrstUpwdDnwdSnsrHmPosLrnd] -> AND14/5
  [SecRwRtStBkReclnUpwdDnwdSnsrHmPosLrnd] -> AND14/6
  [SecRwRtStFrwdBkwdSnsrHmPosLrnd] -> AND14/7
  [SecRwRtStLgrstUpwdDnwdSnsrHmPosLrnd] -> AND14/8
  [SecRwRtStLgrstOtwdInwdSnsrHmPosLrnd] -> AND14/9
  [SecRwRtStCshnFrntUpwdDnwdSnsrHmPosLrnd] -> AND14/10
  [ThdRwLtStCshnFldUpwdDnwdSnsrHmPosLrnd] -> AND14/11
  [ThdRwRtStCshnFldUpwdDnwdSnsrHmPosLrnd] -> AND15/6
  [SecRwRtStCshnFrntUpwdDnwdSnsrHmPosLrnd] -> AND15/5
  [SecRwRtStLgrstOtwdInwdSnsrHmPosLrnd] -> AND15/4
  [SecRwRtStLgrstUpwdDnwdSnsrHmPosLrnd] -> AND15/3
  [SecRwRtStFrwdBkwdSnsrHmPosLrnd] -> AND15/2
  [SecRwRtStBkReclnUpwdDnwdSnsrHmPosLrnd] -> AND15/1
  [SecRwRtStLgrstOtwdInwdSnsrHmPosLrnd] -> AND13/4
  [SecRwRtStLgrstUpwdDnwdSnsrHmPosLrnd] -> AND13/5
  AND21/1 -> Switch89/3
  [KeSMSbIgnorePosLrnd] -> Switch89/2
  Constant68/1 -> Switch89/1
  [PassStBkReclnUpwdDnwdSnsrHmPosLrnd] -> AND21/1
  [PassStFrwdBkwdSnsrHmPosLrnd] -> AND21/2
  [PassStFldUpwdDnwdSnsrHmPosLrnd] -> AND21/3
  [SecRwLtStBkReclnUpwdDnwdSnsrHmPosLrnd] -> AND21/4
  [SecRwLtStFrwdBkwdSnsrHmPosLrnd] -> AND21/5
  [SecRwLtStLgrstUpwdDnwdSnsrHmPosLrnd] -> AND21/6
  [SecRwLtStLgrstOtwdInwdSnsrHmPosLrnd] -> AND21/7
  [SecRwLtStCshnFrntUpwdDnwdSnsrHmPosLrnd] -> AND21/8
  [SecRwRtStLgrstUpwdDnwdSnsrHmPosLrnd] -> AND21/9
  [SecRwRtStFrwdBkwdSnsrHmPosLrnd] -> AND21/10
  [SecRwRtStBkReclnUpwdDnwdSnsrHmPosLrnd] -> AND21/11
  [SecRwRtStLgrstOtwdInwdSnsrHmPosLrnd] -> AND21/12
  [SecRwRtStCshnFrntUpwdDnwdSnsrHmPosLrnd] -> AND21/13
  [ThdRwLtStCshnFldUpwdDnwdSnsrHmPosLrnd] -> Switch90/1
  Equal27/1 -> Switch91/2
  Constant69/1 -> Switch91/3
  Constant71/1 -> Switch90/3
  [IfVeSMSeStNumConfig] -> Equal26/1
  [IfVeSMSeStNumConfig] -> Equal27/1
  Constant70/1 -> Equal26/2
  [ThdRwRtStCshnFldUpwdDnwdSnsrHmPosLrnd] -> Switch91/1
  Equal26/1 -> Switch90/2
  Constant72/1 -> Equal27/2
  Switch91/1 -> AND21/18
  Switch90/1 -> AND21/15
  [ThdRwLtStBkReclnUpwdDnwdSnsrHmPosLrnd] -> AND21/14
  [ThdRwLtStFrwdBkwdSnsrHmPosLrnd] -> AND21/16
  [ThdRwRtStBkReclnUpwdDnwdSnsrHmPosLrnd] -> AND21/17
  [ThdRwRtStFrwdBkwdSnsrHmPosLrnd] -> AND21/19
  Switch89/1 -> IfVeSMSbWholeVehMemPosLrnd_Val_write/1
